simulink model "GeneratorRectifierBuckConverterModel"  (R2021a)
settings: Solver=FixedStepAuto  StartTime=0.0  StopTime=t  FixedStep=tstep  RelTol=1e-3
values from neighbouring files (symbols this model uses):
  buck_catastrophic_fault_toggle = input('   0 = no fault  -or-  1 = fault: ')    [Run_GeneratorRectifierBuckConverterModel.m]
  gen_catastrophic_fault_toggle = input('   0 = no fault  -or-  1 = fault: ')    [Run_GeneratorRectifierBoostConverterInverterMotorModel.m]    (also in Run_GeneratorRectifierBoostConverterModel.m; Run_GeneratorRectifierBuckConverterModel.m; Run_GeneratorRectifierModel.m)
  rect_catastrophic_fault_toggle = input('   0 = no fault  -or-  1 = fault: ')    [Run_GeneratorRectifierBoostConverterInverterMotorModel.m]    (also in Run_GeneratorRectifierBoostConverterModel.m; Run_GeneratorRectifierBuckConverterModel.m; Run_GeneratorRectifierModel.m)
  tstep = 0.001    [Run_GeneratorRectifierBoostConverterInverterMotorModel.m]    (also in Run_GeneratorRectifierBoostConverterModel.m; Run_GeneratorRectifierBuckConverterModel.m; Run_GeneratorRectifierModel.m; Run_InverterMotorModel.m)
undefined symbols (not defined in the file or in its folder): temp
libraries: Lib_EMTAT x3
settings Model: Creator=sfaulk  LastModifiedBy=mebell

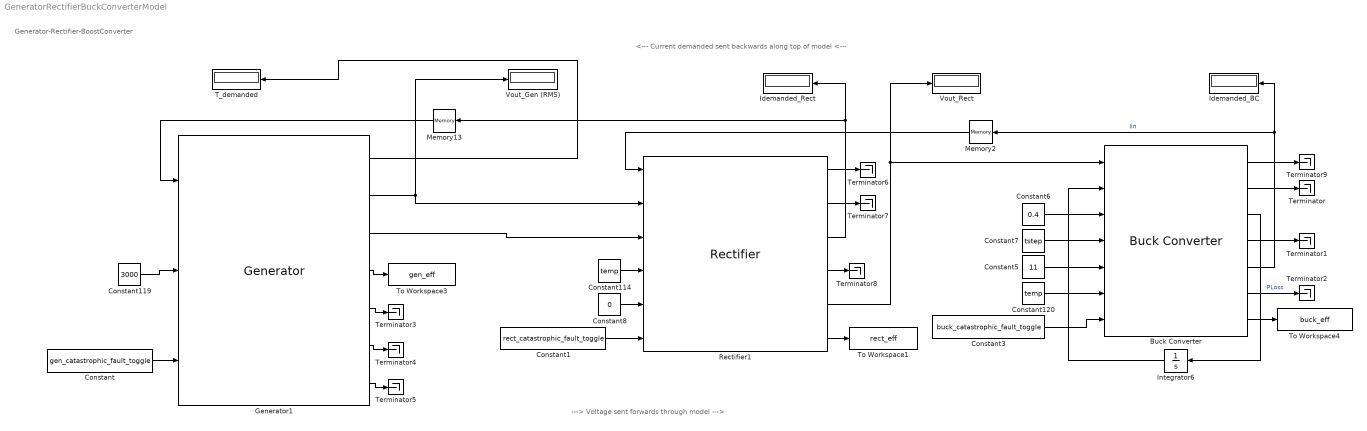
== system GeneratorRectifierBuckConverterModel ==
  note: ---> Voltage sent forwards through model --->
  note: <--- Current demanded sent backwards along top of model <---
  note: Generator-Rectifier-BoostConverter
  Buck Converter : Lib_EMTAT/Components/Physics-Based/Buck Converter  Pdis_M=1  C_M=4.4e-08  L_M=0.0006  Ron_M=0.13  RC_M=0.286  RL_M=0.18923  QgTotal_M=5e-09  Vgate_M=4  TRise_M=2.3e-08  TFall_M=2.2e-08  Fsw_M=250000  Trr_M=2.22e-07  n_MOSFET=1  MassEst_M=0  TempIn=Celsius  vOut=50  pow=100  minV=123  maxV=127  rippleMode=Use defaults (5% of voltage output and 10% of inductor current)  vRip=.05  iRip=.1  freqMode=Use default frequency (250 kHz)  freq=250e3
      settings: SourceProductName=EMTAT
  Constant : Constant  Value=gen_catastrophic_fault_toggle
  Constant1 : Constant  Value=rect_catastrophic_fault_toggle
  Constant114 : Constant  Value=temp
  Constant119 : Constant  Value=3000
  Constant120 : Constant  Value=temp
  Constant3 : Constant  Value=buck_catastrophic_fault_toggle
  Constant5 : Constant  Value=11
  Constant6 : Constant  Value=0.4
  Constant7 : Constant  Value=tstep
  Constant8 : Constant  Value=0
  Generator1 : Lib_EMTAT/Components/Physics-Based/Generator  pp=3  flux_m=0.38515  R_s=0.032  L_s=0.00115  P_Fe_Nom=904.3614  S_nom=4000  T_nom=70  P_out_max=22000  I_max=36.5  P_in_max=30000  T_max=80  MassEst_M=-1080970  Poles_i=6  R_s_i=.032  L_s_i=.00086+0.00029  S_nom_i=4000  T_nom_i=70  P_out_max_i=22000  I_max_i=36.5  P_in_max_i=30000  K_i=121  V_nom_i=368  T_max_i=80  CalculatePFe=Compute iron losses automatically  P_Fe_Nom_i=0  I_nom_i=36.5  PF_nom_i=0.99  P_Fe_Calc_Flag=1
      settings: SourceProductName=EMTAT
  Idemanded_BC : Display
  Idemanded_Rect : Display
  Integrator6 : Integrator
  Memory13 : Memory
  Memory2 : Memory
  Rectifier1 : Lib_EMTAT/Components/Physics-Based/Rectifier  T_M=[25 175]  u_D_M=[1.16666666666667 0.999999999999998]  u_ce0_M=[0.971428571428571 0.848275862068965]  R_c_M=[0.0285714285714286 0.0551724137931034]  R_D_M=[0.0238095238095238 0.0294117647058824]  E0_M=[6.00000000000002e-05 6.00000000000002e-05]  E1_M=[5.6e-05 5.6e-05]  f_sw_M=20000  L_s_M=0.1  P_max_I=22000  V_phase_I=600  f_sw_I=0  L_s_I=0.1
      settings: SourceProductName=EMTAT
  T_demanded : Display
  Terminator{,1..9} (10 alike) : Terminator
  To Workspace1 : ToWorkspace  VariableName=rect_eff  SaveFormat=Timeseries  SampleTime=-1
  To Workspace3 : ToWorkspace  VariableName=gen_eff  SaveFormat=Timeseries  SampleTime=-1
  To Workspace4 : ToWorkspace  VariableName=buck_eff  SaveFormat=Timeseries  SampleTime=-1
  Vout_Gen (RMS) : Display
  Vout_Rect : Display
  wires:
  Rectifier1/6 -> To Workspace1/1
  Rectifier1/1 -> Terminator6/1
  Constant/1 -> Generator1/3
  Generator1/1 -> T_demanded/1
  Buck Converter/6 -> Terminator2/1  "PLoss"
  Rectifier1/5 -> Buck Converter/1, Vout_Rect/1
  Generator1/7 -> Terminator5/1
  Generator1/6 -> Terminator4/1
  Rectifier1/2 -> Terminator7/1
  Generator1/5 -> Terminator3/1
  Rectifier1/4 -> Terminator8/1
  Rectifier1/3 -> Idemanded_Rect/1, Memory13/1
  Integrator6/1 -> Buck Converter/2
  Constant6/1 -> Buck Converter/3
  Constant3/1 -> Buck Converter/7
  Constant8/1 -> Rectifier1/5
  Constant120/1 -> Buck Converter/6
  Generator1/4 -> To Workspace3/1
  Generator1/2 -> Rectifier1/2, Vout_Gen (RMS)/1
  Constant7/1 -> Buck Converter/4
  Generator1/3 -> Rectifier1/3
  Buck Converter/4 -> Terminator1/1
  Constant119/1 -> Generator1/2
  Buck Converter/5 -> Idemanded_BC/1, Memory2/1  "Iin"
  Buck Converter/2 -> Terminator/1
  Memory13/1 -> Generator1/1
  Constant1/1 -> Rectifier1/6
  Memory2/1 -> Rectifier1/1
  Constant114/1 -> Rectifier1/4
  Buck Converter/3 -> Integrator6/1
  Constant5/1 -> Buck Converter/5
  Buck Converter/7 -> To Workspace4/1
  Buck Converter/1 -> Terminator9/1
